simulink model "full_maneuver_platoon"  (R2022a)
settings: Solver=ode23t  StartTime=0.0  StopTime=300  FixedStep=0.1  MaxStep=0.01  RelTol=1e-3
InitFcn:
  | totalVehicles = 7;
  | if exist('vehStatesBus', 'var')==0
  | load vehBuses
  | end
  | if exist('vehErrorsBus', 'var')==0
  | load vehBuses
  | end
libraries: simulink x80, powerlib_meascontrol x16, autolibshared x7, dspsigops x4
(part 8 of 9)

== stateflow chart full_maneuver_platoon/p1/Lane Change Strategy/Strategy 1: synchronous/Chart ==
  state laneKeeping
    entry:
    maneuverState = 0;
    % canStartLaneChange = false;
  state generatingGapForMergingVehicle
    entry:
    maneuverState = 1;
    hasVirtualLeader = true;
  state gapClosing
    entry:
    maneuverState = 5;
    mustIncreaseGap = false;
  state generatingGap
    entry:
    maneuverState = 1;
    mustIncreaseGap = true;
    if positionInPlatoon == 1
    hasVirtualLeader = true;
    end
    if positionInPlatoon == length(platoonStates)
    hasVirtualFollower = true;
    end
  state waitingForGapClosing
    entry:
    maneuverState = 4;
    hasVirtualLeader = false;
  state laneChanging
    entry:
    maneuverState = 3;
    canStartLaneChange = true;
    hasVirtualFollower = false;
  state waitingForPlatoonSafeGap
    entry:
    maneuverState = 2;
  (default) -> laneKeeping
  laneKeeping -> generatingGapForMergingVehicle [order 1] : [gapRequest && platoonStates(end) <= 3]
  generatingGapForMergingVehicle -> laneKeeping : [platoonStates(end) > 3]
  gapClosing -> laneKeeping : [isGapClosed || (positionInPlatoon==1 ...
      | && realCACCstate~=1 && sum(platoonStates(2:end))==0 ...
      | && after(1, sec))]
  laneKeeping -> generatingGap [order 2] : [hasLaneChangeIntention && ~isLaneChangeDone ...
      |  && ((positionInPlatoon == 1) || (platoonStates(positionInPlatoon - 1)>1))]
  waitingForGapClosing -> gapClosing : [positionInPlatoon == length(platoonStates) || ...
      | platoonStates(positionInPlatoon + 1) == 0]
  laneChanging -> waitingForGapClosing : [isLaneChangeDone]
  generatingGap -> waitingForPlatoonSafeGap : [isLaneChangeSafe]
  waitingForPlatoonSafeGap -> laneChanging : [platoonStates(end)>1]
  data: gapRequest input; hasLaneChangeIntention input; maneuverState output uint8 =uint8(0); mustIncreaseGap output =false; positionInPlatoon input; platoonStates input; isLaneChangeDone input; isLaneChangeSafe input; canStartLaneChange output =false; hasVirtualLeader output =false; hasVirtualFollower output =false; isGapClosed input; realCACCstate input

== matlab function full_maneuver_platoon/p1/Lane Change Strategy/Strategy 1: synchronous/determine virtual leader idx/determineVirtualLeader ==
  data: nVehicles input; lcFlag input; virtualLeaderIdx output
function virtualLeaderIdx  = ...
    determineVirtualLeader(nVehicles, lcFlag)

% Strategy 'synchronous': all vehicles move together when gap fits the
% whole platoon
% Important assumption:
% The array of vehicles is ordered as [Ld, Fd, Lo, p1, ..., pN, Fo]

if ~lcFlag % gap generating vehicle
    virtualLeaderIdx = nVehicles-1; % last platoon vehicle
else % lane changing vehicle
    virtualLeaderIdx = 1;
end

end

== stateflow chart full_maneuver_platoon/p1/Lane Change Strategy/Strategy 2: leader first/Chart ==
  state laneKeeping
    entry:
    maneuverState = 0;
    % canStartLaneChange = false;
  state generatingGapForMergingVehicle
    entry:
    maneuverState = 1;
    hasVirtualLeader = true;
  state gapClosing
    entry:
    maneuverState = 5;
    mustIncreaseGap = false;
  state waitingLeaderLaneChange
    entry:
    maneuverState = 1;
    hasVirtualLeader = true;
  state waitingForGapClosing
    entry:
    maneuverState = 4;
    hasVirtualLeader = false;
  state laneChanging
    entry:
    maneuverState = 3;
    canStartLaneChange = true;
    hasVirtualFollower = false;
  state generatingGap
    entry:
    maneuverState = 2;
    mustIncreaseGap = true;
    hasVirtualLeader = true;
    hasVirtualFollower = true;
  (default) -> laneKeeping
  laneKeeping -> generatingGapForMergingVehicle [order 2] : [gapRequest && platoonStates(end) <= 3]
  gapClosing -> laneKeeping : [isGapClosed || (positionInPlatoon==1 ...
      | && realCACCstate~=1 && sum(platoonStates(2:end))==0 ...
      | && after(1, sec))]
  generatingGapForMergingVehicle -> laneKeeping : [platoonStates(end) > 3]
  laneKeeping -> waitingLeaderLaneChange [order 1] : [hasLaneChangeIntention && ~isLaneChangeDone ...
      |  && (positionInPlatoon == 1 || platoonStates(positionInPlatoon - 1) > 1)]
  waitingForGapClosing -> gapClosing : [true]
  waitingLeaderLaneChange -> generatingGap : [positionInPlatoon == 1 || platoonStates(positionInPlatoon - 1) > 4]
  laneChanging -> waitingForGapClosing : [isLaneChangeDone]
  generatingGap -> laneChanging : [isLaneChangeSafe]
  data: gapRequest input; hasLaneChangeIntention input; maneuverState output uint8 =uint8(0); mustIncreaseGap output =false; positionInPlatoon input; platoonStates input; isLaneChangeDone input; isLaneChangeSafe input; canStartLaneChange output =false; hasVirtualLeader output =false; hasVirtualFollower output =false; isGapClosed input; realCACCstate input

== matlab function full_maneuver_platoon/p1/Lane Change Strategy/Strategy 2: leader first/determine virtual leader idx/determineVirtualLeader ==
  data: nVehicles input; lcFlag input; virtualLeaderIdx output; posInPlatoon input
function virtualLeaderIdx  = ...
    determineVirtualLeader(nVehicles, lcFlag, posInPlatoon)

% Strategy: leader changes first 
% Important assumption:
% The array of vehicles is ordered as [Ld, Fd, Lo, p1, ..., pN, Fo]

if ~lcFlag% gap generating vehicle
    virtualLeaderIdx = nVehicles-1; % last platoon vehicle    
else % lane changing vehicle:  
    if posInPlatoon == 1
        virtualLeaderIdx = 1;
    else
        % all platoon vehicles adopt the real leading vehicle as
        % virtual leaders too
        virtualLeaderIdx = 3 + (posInPlatoon - 1);
    end
end

end

== stateflow chart full_maneuver_platoon/p1/Lane Change Strategy/Strategy 3: last first/Chart ==
  state generatingGapForMergingVehicle
    entry:
    maneuverState = 1;
    hasVirtualLeader = true;
  state laneKeeping
    entry:
    maneuverState = 0;
    % canStartLaneChange = false;
  state gapClosing
    entry:
    maneuverState = 5;
    hasVirtualLeader = false;
  state creatingGapForNextVehicle
    entry:
    maneuverState = 4;
    mustIncreaseGap = false;
  state generatingGap
    entry:
    maneuverState = 1;
    mustIncreaseGap = true;
    hasVirtualLeader = true;
    hasVirtualFollower = true;
  state laneChanging
    entry:
    maneuverState = 3;
    canStartLaneChange = true;
    hasVirtualFollower = false;
  (default) -> laneKeeping
  gapClosing -> laneKeeping : [isGapClosed || (positionInPlatoon==1 ...
      | && realCACCstate~=1 && sum(platoonStates(2:end))==0 ...
      | && after(1, sec))]
  laneKeeping -> generatingGapForMergingVehicle [order 2] : [gapRequest && platoonStates(end) <= 3]
  generatingGapForMergingVehicle -> laneKeeping : [platoonStates(end) > 3]
  laneKeeping -> generatingGap [order 1] : [hasLaneChangeIntention && ~isLaneChangeDone ...
      |  && (positionInPlatoon == length(platoonStates) || platoonStates(positionInPlatoon + 1) > 3)]
  creatingGapForNextVehicle -> gapClosing : [positionInPlatoon == 1 || ...
      | platoonStates(positionInPlatoon - 1) > 3]
  laneChanging -> creatingGapForNextVehicle : [isLaneChangeDone]
  generatingGap -> laneChanging : [isLaneChangeSafe]
  data: gapRequest input; hasLaneChangeIntention input; maneuverState output uint8 =uint8(0); mustIncreaseGap output =false; positionInPlatoon input; platoonStates input; isLaneChangeDone input; isLaneChangeSafe input; canStartLaneChange output =false; hasVirtualLeader output =false; hasVirtualFollower output =false; isGapClosed input; realCACCstate input

== matlab function full_maneuver_platoon/p1/Lane Change Strategy/Strategy 3: last first/determine virtual follower idx/determineVirtualFollower ==
  data: platoonSize input; posInPlatoon input; virtualFollowerIdx output
function virtualFollowerIdx  = ...
    determineVirtualFollower(platoonSize, posInPlatoon)

% Strategy 'lastFirst': last veh changes first and creates gap for leader
% Important assumption:
% The array of vehicles is ordered as [Ld, Fd, Lo, p1, ..., pN, Fo]

if posInPlatoon == platoonSize
    virtualFollowerIdx = 2;
else
    virtualFollowerIdx = 3 + (posInPlatoon + 1);
end

end

== matlab function full_maneuver_platoon/p1/Lane Change Strategy/Strategy 3: last first/determine virtual leader idx/determineVirtualLeader ==
  data: nVehicles input; lcFlag input; lcDone input; virtualLeaderIdx output; posInPlatoon input
function virtualLeaderIdx  = ...
    determineVirtualLeader(nVehicles, lcFlag, lcDone, posInPlatoon)

% Strategy 'lastFirst': last veh changes first and creates gap for leader
% Important assumption:
% The array of vehicles is ordered as [Ld, Fd, Lo, p1, ..., pN, Fo]

if ~lcFlag% gap generating vehicle
    virtualLeaderIdx = nVehicles-1; % last platoon vehicle
else % lane changing vehicle
    if ~lcDone
        virtualLeaderIdx = 1;
    else
        if posInPlatoon == 1
            virtualLeaderIdx = 1;
        else
            virtualLeaderIdx = 3 + (posInPlatoon - 1);
        end
    end
    
end

end

== stateflow chart full_maneuver_platoon/p1/Lane Change Strategy/Strategy 4: leader first invert/Chart ==
  state laneKeeping
    entry:
    maneuverState = 0;
    % canStartLaneChange = false;
  state generatingGapForMergingVehicle
    entry:
    maneuverState = 1;
    hasVirtualLeader = true;
  state gapClosing
    entry:
    maneuverState = 5;
    hasVirtualLeader = false;
  state creatingGapForNextVehicle
    entry:
    maneuverState = 4;
    mustIncreaseGap = false;
  state generatingGap
    entry:
    maneuverState = 1;
    mustIncreaseGap = true;
    hasVirtualLeader = true;
    hasVirtualFollower = true;
  state laneChanging
    entry:
    maneuverState = 3;
    canStartLaneChange = true;
    hasVirtualFollower = false;
  (default) -> laneKeeping
  gapClosing -> laneKeeping : [isGapClosed || (positionInPlatoon==length(platoonStates)...
      | && realCACCstate~=1 && sum(platoonStates(1:end-1))==0 ...
      | && after(1, sec))]
  laneKeeping -> generatingGapForMergingVehicle [order 2] : [gapRequest && platoonStates(1) <= 3]
  generatingGapForMergingVehicle -> laneKeeping : [platoonStates(1) > 3]
  laneKeeping -> generatingGap [order 1] : [hasLaneChangeIntention && ~isLaneChangeDone ...
      |  && (positionInPlatoon == 1 || platoonStates(positionInPlatoon - 1) > 3)]
  creatingGapForNextVehicle -> gapClosing : [positionInPlatoon == length(platoonStates) || ...
      | platoonStates(positionInPlatoon + 1) > 3]
  laneChanging -> creatingGapForNextVehicle : [isLaneChangeDone]
  generatingGap -> laneChanging : [isLaneChangeSafe]
  data: gapRequest input; hasLaneChangeIntention input; maneuverState output uint8 =uint8(0); mustIncreaseGap output =false; positionInPlatoon input; platoonStates input; isLaneChangeDone input; isLaneChangeSafe input; canStartLaneChange output =false; hasVirtualLeader output =false; hasVirtualFollower output =false; isGapClosed input; realCACCstate input

== matlab function full_maneuver_platoon/p1/Lane Change Strategy/Strategy 4: leader first invert/Subsystem/determineVirtualFollower ==
  data: posInPlatoon input; virtualFollowerIdx output
function virtualFollowerIdx  = ...
    determineVirtualFollower(posInPlatoon)

% Strategy 'leaderFirstInvert': leader changes first and creates gap for 
%next
% Important assumption:
% The array of vehicles is ordered as [Ld, Fd, Lo, p1, ..., pN, Fo]

if posInPlatoon == 1
    virtualFollowerIdx = 2;
else
    virtualFollowerIdx = 3 + (posInPlatoon - 1);
end


end

== matlab function full_maneuver_platoon/p1/Lane Change Strategy/Strategy 4: leader first invert/Subsystem1/determineVirtualLeader ==
  data: nVehicles input; lcFlag input; lcDone input; virtualLeaderIdx output; posInPlatoon input
function virtualLeaderIdx  = ...
    determineVirtualLeader(nVehicles, lcFlag, lcDone, posInPlatoon)

% Strategy 'leaderFirstInvert': leader changes first and creates gap for 
%next
% Important assumption:
% The array of vehicles is ordered as [Ld, Fd, Lo, p1, ..., pN, Fo]

platoonLength = nVehicles - 4;
if ~lcFlag% gap generating vehicle
    virtualLeaderIdx = 4; % first platoon vehicle
else % lane changing vehicle
    if ~lcDone
        virtualLeaderIdx = 1;
    else
        if posInPlatoon == platoonLength
            virtualLeaderIdx = 1;
        else
            virtualLeaderIdx = 3 + (posInPlatoon + 1);
        end
    end
end

end

== matlab function full_maneuver_platoon/p2/CACC destination lane/Virtual Vehicle Following/switch min vel/MATLAB Function ==
  data: h input; maxGap output; d0 input; vRef input; ev input; ehDot input; ea input; Kp parameter; Kd parameter; Ka parameter; Kdd parameter
function maxGap = followingGapThreshold(h, d0, vRef, ev, ehDot, ea, Kp, Kd, Ka, Kdd)

maxGap = h*vRef + d0 - 1/Kp*(Kd*ev + Kdd*ehDot + Ka*ea);

== matlab function full_maneuver_platoon/p2/CACC origin lane/switch free flow/MATLAB Function ==
  data: h input; maxGap output; d0 input; vRef input; ev input; ehDot input; ea input; Kp parameter; Kd parameter; Ka parameter; Kdd parameter
function maxGap = followingGapThreshold(h, d0, vRef, ev, ehDot, ea, Kp, Kd, Ka, Kdd)

maxGap = h*vRef + d0 - 1/Kp*(Kd*ev + Kdd*ehDot + Ka*ea);

== matlab function full_maneuver_platoon/p2/Find Leader/Subsystem/MATLAB Function ==
  data: ego input Bus: vehStatesBus; allVehicles input; leaderIdx output
function leaderIdx  = findLeader(ego, allVehicles)

nv = length(allVehicles);

leaderIdx = nv + 1;
leaderX = ego.X + 10^3;
% For non lane changing vehicles, the leader is whoever is longitudinally
% closer and with any part of the body in the same lane.
% 1.8m (half lane) + 0.9m (half veh width)
for n = 1:nv
    if allVehicles(n).X > ego.X
        if abs(allVehicles(n).Y - ego.Y) <= 2.7 ...
                && allVehicles(n).X < leaderX
            leaderIdx = n;
            leaderX = allVehicles(n).X;
        end
    end
end

== stateflow chart full_maneuver_platoon/p2/Lane Change Strategy/Strategy 1: synchronous/Chart ==
  state laneKeeping
    entry:
    maneuverState = 0;
    % canStartLaneChange = false;
  state generatingGapForMergingVehicle
    entry:
    maneuverState = 1;
    hasVirtualLeader = true;
  state gapClosing
    entry:
    maneuverState = 5;
    mustIncreaseGap = false;
  state generatingGap
    entry:
    maneuverState = 1;
    mustIncreaseGap = true;
    if positionInPlatoon == 1
    hasVirtualLeader = true;
    end
    if positionInPlatoon == length(platoonStates)
    hasVirtualFollower = true;
    end
  state waitingForGapClosing
    entry:
    maneuverState = 4;
    hasVirtualLeader = false;
  state laneChanging
    entry:
    maneuverState = 3;
    canStartLaneChange = true;
    hasVirtualFollower = false;
  state waitingForPlatoonSafeGap
    entry:
    maneuverState = 2;
  (default) -> laneKeeping
  laneKeeping -> generatingGapForMergingVehicle [order 1] : [gapRequest && platoonStates(end) <= 3]
  generatingGapForMergingVehicle -> laneKeeping : [platoonStates(end) > 3]
  gapClosing -> laneKeeping : [isGapClosed || (positionInPlatoon==1 ...
      | && realCACCstate~=1 && sum(platoonStates(2:end))==0 ...
      | && after(1, sec))]
  laneKeeping -> generatingGap [order 2] : [hasLaneChangeIntention && ~isLaneChangeDone ...
      |  && ((positionInPlatoon == 1) || (platoonStates(positionInPlatoon - 1)>1))]
  waitingForGapClosing -> gapClosing : [positionInPlatoon == length(platoonStates) || ...
      | platoonStates(positionInPlatoon + 1) == 0]
  laneChanging -> waitingForGapClosing : [isLaneChangeDone]
  generatingGap -> waitingForPlatoonSafeGap : [isLaneChangeSafe]
  waitingForPlatoonSafeGap -> laneChanging : [platoonStates(end)>1]
  data: gapRequest input; hasLaneChangeIntention input; maneuverState output uint8 =uint8(0); mustIncreaseGap output =false; positionInPlatoon input; platoonStates input; isLaneChangeDone input; isLaneChangeSafe input; canStartLaneChange output =false; hasVirtualLeader output =false; hasVirtualFollower output =false; isGapClosed input; realCACCstate input

== matlab function full_maneuver_platoon/p2/Lane Change Strategy/Strategy 1: synchronous/determine virtual leader idx/determineVirtualLeader ==
  data: nVehicles input; lcFlag input; virtualLeaderIdx output
function virtualLeaderIdx  = ...
    determineVirtualLeader(nVehicles, lcFlag)

% Strategy 'synchronous': all vehicles move together when gap fits the
% whole platoon
% Important assumption:
% The array of vehicles is ordered as [Ld, Fd, Lo, p1, ..., pN, Fo]

if ~lcFlag % gap generating vehicle
    virtualLeaderIdx = nVehicles-1; % last platoon vehicle
else % lane changing vehicle
    virtualLeaderIdx = 1;
end

end

== stateflow chart full_maneuver_platoon/p2/Lane Change Strategy/Strategy 2: leader first/Chart ==
  state laneKeeping
    entry:
    maneuverState = 0;
    % canStartLaneChange = false;
  state generatingGapForMergingVehicle
    entry:
    maneuverState = 1;
    hasVirtualLeader = true;
  state gapClosing
    entry:
    maneuverState = 5;
    mustIncreaseGap = false;
  state waitingLeaderLaneChange
    entry:
    maneuverState = 1;
    hasVirtualLeader = true;
  state waitingForGapClosing
    entry:
    maneuverState = 4;
    hasVirtualLeader = false;
  state laneChanging
    entry:
    maneuverState = 3;
    canStartLaneChange = true;
    hasVirtualFollower = false;
  state generatingGap
    entry:
    maneuverState = 2;
    mustIncreaseGap = true;
    hasVirtualLeader = true;
    hasVirtualFollower = true;
  (default) -> laneKeeping
  laneKeeping -> generatingGapForMergingVehicle [order 2] : [gapRequest && platoonStates(end) <= 3]
  gapClosing -> laneKeeping : [isGapClosed || (positionInPlatoon==1 ...
      | && realCACCstate~=1 && sum(platoonStates(2:end))==0 ...
      | && after(1, sec))]
  generatingGapForMergingVehicle -> laneKeeping : [platoonStates(end) > 3]
  laneKeeping -> waitingLeaderLaneChange [order 1] : [hasLaneChangeIntention && ~isLaneChangeDone ...
      |  && (positionInPlatoon == 1 || platoonStates(positionInPlatoon - 1) > 1)]
  waitingForGapClosing -> gapClosing : [true]
  waitingLeaderLaneChange -> generatingGap : [positionInPlatoon == 1 || platoonStates(positionInPlatoon - 1) > 4]
  laneChanging -> waitingForGapClosing : [isLaneChangeDone]
  generatingGap -> laneChanging : [isLaneChangeSafe]
  data: gapRequest input; hasLaneChangeIntention input; maneuverState output uint8 =uint8(0); mustIncreaseGap output =false; positionInPlatoon input; platoonStates input; isLaneChangeDone input; isLaneChangeSafe input; canStartLaneChange output =false; hasVirtualLeader output =false; hasVirtualFollower output =false; isGapClosed input; realCACCstate input

== matlab function full_maneuver_platoon/p2/Lane Change Strategy/Strategy 2: leader first/determine virtual leader idx/determineVirtualLeader ==
  data: nVehicles input; lcFlag input; virtualLeaderIdx output; posInPlatoon input
function virtualLeaderIdx  = ...
    determineVirtualLeader(nVehicles, lcFlag, posInPlatoon)

% Strategy: leader changes first 
% Important assumption:
% The array of vehicles is ordered as [Ld, Fd, Lo, p1, ..., pN, Fo]

if ~lcFlag% gap generating vehicle
    virtualLeaderIdx = nVehicles-1; % last platoon vehicle    
else % lane changing vehicle:  
    if posInPlatoon == 1
        virtualLeaderIdx = 1;
    else
        % all platoon vehicles adopt the real leading vehicle as
        % virtual leaders too
        virtualLeaderIdx = 3 + (posInPlatoon - 1);
    end
end

end

== stateflow chart full_maneuver_platoon/p2/Lane Change Strategy/Strategy 3: last first/Chart ==
  state generatingGapForMergingVehicle
    entry:
    maneuverState = 1;
    hasVirtualLeader = true;
  state laneKeeping
    entry:
    maneuverState = 0;
    % canStartLaneChange = false;
  state gapClosing
    entry:
    maneuverState = 5;
    hasVirtualLeader = false;
  state creatingGapForNextVehicle
    entry:
    maneuverState = 4;
    mustIncreaseGap = false;
  state generatingGap
    entry:
    maneuverState = 1;
    mustIncreaseGap = true;
    hasVirtualLeader = true;
    hasVirtualFollower = true;
  state laneChanging
    entry:
    maneuverState = 3;
    canStartLaneChange = true;
    hasVirtualFollower = false;
  (default) -> laneKeeping
  gapClosing -> laneKeeping : [isGapClosed || (positionInPlatoon==1 ...
      | && realCACCstate~=1 && sum(platoonStates(2:end))==0 ...
      | && after(1, sec))]
  laneKeeping -> generatingGapForMergingVehicle [order 2] : [gapRequest && platoonStates(end) <= 3]
  generatingGapForMergingVehicle -> laneKeeping : [platoonStates(end) > 3]
  laneKeeping -> generatingGap [order 1] : [hasLaneChangeIntention && ~isLaneChangeDone ...
      |  && (positionInPlatoon == length(platoonStates) || platoonStates(positionInPlatoon + 1) > 3)]
  creatingGapForNextVehicle -> gapClosing : [positionInPlatoon == 1 || ...
      | platoonStates(positionInPlatoon - 1) > 3]
  laneChanging -> creatingGapForNextVehicle : [isLaneChangeDone]
  generatingGap -> laneChanging : [isLaneChangeSafe]
  data: gapRequest input; hasLaneChangeIntention input; maneuverState output uint8 =uint8(0); mustIncreaseGap output =false; positionInPlatoon input; platoonStates input; isLaneChangeDone input; isLaneChangeSafe input; canStartLaneChange output =false; hasVirtualLeader output =false; hasVirtualFollower output =false; isGapClosed input; realCACCstate input

== matlab function full_maneuver_platoon/Lo/CACC origin lane/Controller Real Leader/switch free flow/MATLAB Function ==
  data: h input; maxGap output; d0 input; vRef input; ev input; ehDot input; ea input; Kp parameter; Kd parameter; Ka parameter; Kdd parameter
function maxGap = followingGapThreshold(h, d0, vRef, ev, ehDot, ea, Kp, Kd, Ka, Kdd)

maxGap = h*vRef + d0 - 1/Kp*(Kd*ev + Kdd*ehDot + Ka*ea);

== matlab function full_maneuver_platoon/Ld/findLeader/Subsystem/MATLAB Function ==
  data: ego input Bus: vehStatesBus; allVehicles input; leaderIdx output
function leaderIdx  = findLeader(ego, allVehicles)

nv = length(allVehicles);

leaderIdx = nv + 1;
leaderX = ego.X + 10^3;
% For non lane changing vehicles, the leader is whoever is longitudinally
% closer and with any part of the body in the same lane.
% 1.8m (half lane) + 0.9m (half veh width)
for n = 1:nv
    if allVehicles(n).X>ego.X
        if abs(allVehicles(n).Y - ego.Y)<=2.7 && allVehicles(n).X<leaderX
            leaderIdx = n;
            leaderX = allVehicles(n).X;
        end
    end
end

== matlab function full_maneuver_platoon/Lo/findLeader/Subsystem/MATLAB Function ==
  data: ego input Bus: vehStatesBus; allVehicles input; leaderIdx output
function leaderIdx  = findLeader(ego, allVehicles)

nv = length(allVehicles);

leaderIdx = nv + 1;
leaderX = ego.X + 10^3;
% For non lane changing vehicles, the leader is whoever is longitudinally
% closer and with any part of the body in the same lane.
% 1.8m (half lane) + 0.9m (half veh width)
for n = 1:nv
    if allVehicles(n).X>ego.X
        if abs(allVehicles(n).Y - ego.Y)<=2.7 && allVehicles(n).X<leaderX
            leaderIdx = n;
            leaderX = allVehicles(n).X;
        end
    end
end

== matlab function full_maneuver_platoon/p2/Lane Change Strategy/Strategy 3: last first/determine virtual follower idx/determineVirtualFollower ==
  data: platoonSize input; posInPlatoon input; virtualFollowerIdx output
function virtualFollowerIdx  = ...
    determineVirtualFollower(platoonSize, posInPlatoon)

% Strategy 'lastFirst': last veh changes first and creates gap for leader
% Important assumption:
% The array of vehicles is ordered as [Ld, Fd, Lo, p1, ..., pN, Fo]

if posInPlatoon == platoonSize
    virtualFollowerIdx = 2;
else
    virtualFollowerIdx = 3 + (posInPlatoon + 1);
end

end

== matlab function full_maneuver_platoon/p1/CACC destination lane/Virtual Vehicle Following/switch min vel/MATLAB Function ==
  data: h input; maxGap output; d0 input; vRef input; ev input; ehDot input; ea input; Kp parameter; Kd parameter; Ka parameter; Kdd parameter
function maxGap = followingGapThreshold(h, d0, vRef, ev, ehDot, ea, Kp, Kd, Ka, Kdd)

maxGap = h*vRef + d0 - 1/Kp*(Kd*ev + Kdd*ehDot + Ka*ea);

== matlab function full_maneuver_platoon/p2/Lane Change Strategy/Strategy 3: last first/determine virtual leader idx/determineVirtualLeader ==
  data: nVehicles input; lcFlag input; lcDone input; virtualLeaderIdx output; posInPlatoon input
function virtualLeaderIdx  = ...
    determineVirtualLeader(nVehicles, lcFlag, lcDone, posInPlatoon)

% Strategy 'lastFirst': last veh changes first and creates gap for leader
% Important assumption:
% The array of vehicles is ordered as [Ld, Fd, Lo, p1, ..., pN, Fo]

if ~lcFlag% gap generating vehicle
    virtualLeaderIdx = nVehicles-1; % last platoon vehicle
else % lane changing vehicle
    if ~lcDone
        virtualLeaderIdx = 1;
    else
        if posInPlatoon == 1
            virtualLeaderIdx = 1;
        else
            virtualLeaderIdx = 3 + (posInPlatoon - 1);
        end
    end
    
end

end

== stateflow chart full_maneuver_platoon/p2/Lane Change Strategy/Strategy 4: leader first invert/Chart ==
  state laneKeeping
    entry:
    maneuverState = 0;
    % canStartLaneChange = false;
  state generatingGapForMergingVehicle
    entry:
    maneuverState = 1;
    hasVirtualLeader = true;
  state gapClosing
    entry:
    maneuverState = 5;
    hasVirtualLeader = false;
  state creatingGapForNextVehicle
    entry:
    maneuverState = 4;
    mustIncreaseGap = false;
  state generatingGap
    entry:
    maneuverState = 1;
    mustIncreaseGap = true;
    hasVirtualLeader = true;
    hasVirtualFollower = true;
  state laneChanging
    entry:
    maneuverState = 3;
    canStartLaneChange = true;
    hasVirtualFollower = false;
  (default) -> laneKeeping
  gapClosing -> laneKeeping : [isGapClosed || (positionInPlatoon==length(platoonStates)...
      | && realCACCstate~=1 && sum(platoonStates(1:end-1))==0 ...
      | && after(1, sec))]
  laneKeeping -> generatingGapForMergingVehicle [order 2] : [gapRequest && platoonStates(1) <= 3]
  generatingGapForMergingVehicle -> laneKeeping : [platoonStates(1) > 3]
  laneKeeping -> generatingGap [order 1] : [hasLaneChangeIntention && ~isLaneChangeDone ...
      |  && (positionInPlatoon == 1 || platoonStates(positionInPlatoon - 1) > 3)]
  creatingGapForNextVehicle -> gapClosing : [positionInPlatoon == length(platoonStates) || ...
      | platoonStates(positionInPlatoon + 1) > 3]
  laneChanging -> creatingGapForNextVehicle : [isLaneChangeDone]
  generatingGap -> laneChanging : [isLaneChangeSafe]
  data: gapRequest input; hasLaneChangeIntention input; maneuverState output uint8 =uint8(0); mustIncreaseGap output =false; positionInPlatoon input; platoonStates input; isLaneChangeDone input; isLaneChangeSafe input; canStartLaneChange output =false; hasVirtualLeader output =false; hasVirtualFollower output =false; isGapClosed input; realCACCstate input

== matlab function full_maneuver_platoon/p2/Lane Change Strategy/Strategy 4: leader first invert/Subsystem/determineVirtualFollower ==
  data: posInPlatoon input; virtualFollowerIdx output
function virtualFollowerIdx  = ...
    determineVirtualFollower(posInPlatoon)

% Strategy 'leaderFirstInvert': leader changes first and creates gap for 
%next
% Important assumption:
% The array of vehicles is ordered as [Ld, Fd, Lo, p1, ..., pN, Fo]

if posInPlatoon == 1
    virtualFollowerIdx = 2;
else
    virtualFollowerIdx = 3 + (posInPlatoon - 1);
end


end

== matlab function full_maneuver_platoon/p2/Lane Change Strategy/Strategy 4: leader first invert/Subsystem1/determineVirtualLeader ==
  data: nVehicles input; lcFlag input; lcDone input; virtualLeaderIdx output; posInPlatoon input
function virtualLeaderIdx  = ...
    determineVirtualLeader(nVehicles, lcFlag, lcDone, posInPlatoon)

% Strategy 'leaderFirstInvert': leader changes first and creates gap for 
%next
% Important assumption:
% The array of vehicles is ordered as [Ld, Fd, Lo, p1, ..., pN, Fo]

platoonLength = nVehicles - 4;
if ~lcFlag% gap generating vehicle
    virtualLeaderIdx = 4; % first platoon vehicle
else % lane changing vehicle
    if ~lcDone
        virtualLeaderIdx = 1;
    else
        if posInPlatoon == platoonLength
            virtualLeaderIdx = 1;
        else
            virtualLeaderIdx = 3 + (posInPlatoon + 1);
        end
    end
end

end

== matlab function full_maneuver_platoon/p3/CACC destination lane/Virtual Vehicle Following/switch min vel/MATLAB Function ==
  data: h input; maxGap output; d0 input; vRef input; ev input; ehDot input; ea input; Kp parameter; Kd parameter; Ka parameter; Kdd parameter
function maxGap = followingGapThreshold(h, d0, vRef, ev, ehDot, ea, Kp, Kd, Ka, Kdd)

maxGap = h*vRef + d0 - 1/Kp*(Kd*ev + Kdd*ehDot + Ka*ea);

== matlab function full_maneuver_platoon/p3/CACC origin lane/switch free flow/MATLAB Function ==
  data: h input; maxGap output; d0 input; vRef input; ev input; ehDot input; ea input; Kp parameter; Kd parameter; Ka parameter; Kdd parameter
function maxGap = followingGapThreshold(h, d0, vRef, ev, ehDot, ea, Kp, Kd, Ka, Kdd)

maxGap = h*vRef + d0 - 1/Kp*(Kd*ev + Kdd*ehDot + Ka*ea);

== matlab function full_maneuver_platoon/p3/Find Leader/Subsystem/MATLAB Function ==
  data: ego input Bus: vehStatesBus; allVehicles input; leaderIdx output
function leaderIdx  = findLeader(ego, allVehicles)

nv = length(allVehicles);

leaderIdx = nv + 1;
leaderX = ego.X + 10^3;
% For non lane changing vehicles, the leader is whoever is longitudinally
% closer and with any part of the body in the same lane.
% 1.8m (half lane) + 0.9m (half veh width)
for n = 1:nv
    if allVehicles(n).X > ego.X
        if abs(allVehicles(n).Y - ego.Y) <= 2.7 ...
                && allVehicles(n).X < leaderX
            leaderIdx = n;
            leaderX = allVehicles(n).X;
        end
    end
end

== stateflow chart full_maneuver_platoon/p3/Lane Change Strategy/Strategy 1: synchronous/Chart ==
  state laneKeeping
    entry:
    maneuverState = 0;
    % canStartLaneChange = false;
  state generatingGapForMergingVehicle
    entry:
    maneuverState = 1;
    hasVirtualLeader = true;
  state gapClosing
    entry:
    maneuverState = 5;
    mustIncreaseGap = false;
  state generatingGap
    entry:
    maneuverState = 1;
    mustIncreaseGap = true;
    if positionInPlatoon == 1
    hasVirtualLeader = true;
    end
    if positionInPlatoon == length(platoonStates)
    hasVirtualFollower = true;
    end
  state waitingForGapClosing
    entry:
    maneuverState = 4;
    hasVirtualLeader = false;
  state laneChanging
    entry:
    maneuverState = 3;
    canStartLaneChange = true;
    hasVirtualFollower = false;
  state waitingForPlatoonSafeGap
    entry:
    maneuverState = 2;
  (default) -> laneKeeping
  laneKeeping -> generatingGapForMergingVehicle [order 1] : [gapRequest && platoonStates(end) <= 3]
  generatingGapForMergingVehicle -> laneKeeping : [platoonStates(end) > 3]
  gapClosing -> laneKeeping : [isGapClosed || (positionInPlatoon==1 ...
      | && realCACCstate~=1 && sum(platoonStates(2:end))==0 ...
      | && after(1, sec))]
  laneKeeping -> generatingGap [order 2] : [hasLaneChangeIntention && ~isLaneChangeDone ...
      |  && ((positionInPlatoon == 1) || (platoonStates(positionInPlatoon - 1)>1))]
  waitingForGapClosing -> gapClosing : [positionInPlatoon == length(platoonStates) || ...
      | platoonStates(positionInPlatoon + 1) == 0]
  laneChanging -> waitingForGapClosing : [isLaneChangeDone]
  generatingGap -> waitingForPlatoonSafeGap : [isLaneChangeSafe]
  waitingForPlatoonSafeGap -> laneChanging : [platoonStates(end)>1]
  data: gapRequest input; hasLaneChangeIntention input; maneuverState output uint8 =uint8(0); mustIncreaseGap output =false; positionInPlatoon input; platoonStates input; isLaneChangeDone input; isLaneChangeSafe input; canStartLaneChange output =false; hasVirtualLeader output =false; hasVirtualFollower output =false; isGapClosed input; realCACCstate input

== matlab function full_maneuver_platoon/Fo/CACC origin lane/Controller Real Leader/switch free flow/MATLAB Function ==
  data: h input; maxGap output; d0 input; vRef input; ev input; ehDot input; ea input; Kp parameter; Kd parameter; Ka parameter; Kdd parameter
function maxGap = followingGapThreshold(h, d0, vRef, ev, ehDot, ea, Kp, Kd, Ka, Kdd)

maxGap = h*vRef + d0 - 1/Kp*(Kd*ev + Kdd*ehDot + Ka*ea);

== matlab function full_maneuver_platoon/p3/Lane Change Strategy/Strategy 1: synchronous/determine virtual leader idx/determineVirtualLeader ==
  data: nVehicles input; lcFlag input; virtualLeaderIdx output
function virtualLeaderIdx  = ...
    determineVirtualLeader(nVehicles, lcFlag)

% Strategy 'synchronous': all vehicles move together when gap fits the
% whole platoon
% Important assumption:
% The array of vehicles is ordered as [Ld, Fd, Lo, p1, ..., pN, Fo]

if ~lcFlag % gap generating vehicle
    virtualLeaderIdx = nVehicles-1; % last platoon vehicle
else % lane changing vehicle
    virtualLeaderIdx = 1;
end

end

== stateflow chart full_maneuver_platoon/p3/Lane Change Strategy/Strategy 2: leader first/Chart ==
  state laneKeeping
    entry:
    maneuverState = 0;
    % canStartLaneChange = false;
  state generatingGapForMergingVehicle
    entry:
    maneuverState = 1;
    hasVirtualLeader = true;
  state gapClosing
    entry:
    maneuverState = 5;
    mustIncreaseGap = false;
  state waitingLeaderLaneChange
    entry:
    maneuverState = 1;
    hasVirtualLeader = true;
  state waitingForGapClosing
    entry:
    maneuverState = 4;
    hasVirtualLeader = false;
  state laneChanging
    entry:
    maneuverState = 3;
    canStartLaneChange = true;
    hasVirtualFollower = false;
  state generatingGap
    entry:
    maneuverState = 2;
    mustIncreaseGap = true;
    hasVirtualLeader = true;
    hasVirtualFollower = true;
  (default) -> laneKeeping
  laneKeeping -> generatingGapForMergingVehicle [order 2] : [gapRequest && platoonStates(end) <= 3]
  gapClosing -> laneKeeping : [isGapClosed || (positionInPlatoon==1 ...
      | && realCACCstate~=1 && sum(platoonStates(2:end))==0 ...
      | && after(1, sec))]
  generatingGapForMergingVehicle -> laneKeeping : [platoonStates(end) > 3]
  laneKeeping -> waitingLeaderLaneChange [order 1] : [hasLaneChangeIntention && ~isLaneChangeDone ...
      |  && (positionInPlatoon == 1 || platoonStates(positionInPlatoon - 1) > 1)]
  waitingForGapClosing -> gapClosing : [true]
  waitingLeaderLaneChange -> generatingGap : [positionInPlatoon == 1 || platoonStates(positionInPlatoon - 1) > 4]
  laneChanging -> waitingForGapClosing : [isLaneChangeDone]
  generatingGap -> laneChanging : [isLaneChangeSafe]
  data: gapRequest input; hasLaneChangeIntention input; maneuverState output uint8 =uint8(0); mustIncreaseGap output =false; positionInPlatoon input; platoonStates input; isLaneChangeDone input; isLaneChangeSafe input; canStartLaneChange output =false; hasVirtualLeader output =false; hasVirtualFollower output =false; isGapClosed input; realCACCstate input

== matlab function full_maneuver_platoon/p1/CACC origin lane/switch free flow/MATLAB Function ==
  data: h input; maxGap output; d0 input; vRef input; ev input; ehDot input; ea input; Kp parameter; Kd parameter; Ka parameter; Kdd parameter
function maxGap = followingGapThreshold(h, d0, vRef, ev, ehDot, ea, Kp, Kd, Ka, Kdd)

maxGap = h*vRef + d0 - 1/Kp*(Kd*ev + Kdd*ehDot + Ka*ea);

== matlab function full_maneuver_platoon/p3/Lane Change Strategy/Strategy 2: leader first/determine virtual leader idx/determineVirtualLeader ==
  data: nVehicles input; lcFlag input; virtualLeaderIdx output; posInPlatoon input
function virtualLeaderIdx  = ...
    determineVirtualLeader(nVehicles, lcFlag, posInPlatoon)

% Strategy: leader changes first 
% Important assumption:
% The array of vehicles is ordered as [Ld, Fd, Lo, p1, ..., pN, Fo]

if ~lcFlag% gap generating vehicle
    virtualLeaderIdx = nVehicles-1; % last platoon vehicle    
else % lane changing vehicle:  
    if posInPlatoon == 1
        virtualLeaderIdx = 1;
    else
        % all platoon vehicles adopt the real leading vehicle as
        % virtual leaders too
        virtualLeaderIdx = 3 + (posInPlatoon - 1);
    end
end

end

== stateflow chart full_maneuver_platoon/p3/Lane Change Strategy/Strategy 3: last first/Chart ==
  state generatingGapForMergingVehicle
    entry:
    maneuverState = 1;
    hasVirtualLeader = true;
  state laneKeeping
    entry:
    maneuverState = 0;
    % canStartLaneChange = false;
  state gapClosing
    entry:
    maneuverState = 5;
    hasVirtualLeader = false;
  state creatingGapForNextVehicle
    entry:
    maneuverState = 4;
    mustIncreaseGap = false;
  state generatingGap
    entry:
    maneuverState = 1;
    mustIncreaseGap = true;
    hasVirtualLeader = true;
    hasVirtualFollower = true;
  state laneChanging
    entry:
    maneuverState = 3;
    canStartLaneChange = true;
    hasVirtualFollower = false;
  (default) -> laneKeeping
  gapClosing -> laneKeeping : [isGapClosed || (positionInPlatoon==1 ...
      | && realCACCstate~=1 && sum(platoonStates(2:end))==0 ...
      | && after(1, sec))]
  laneKeeping -> generatingGapForMergingVehicle [order 2] : [gapRequest && platoonStates(end) <= 3]
  generatingGapForMergingVehicle -> laneKeeping : [platoonStates(end) > 3]
  laneKeeping -> generatingGap [order 1] : [hasLaneChangeIntention && ~isLaneChangeDone ...
      |  && (positionInPlatoon == length(platoonStates) || platoonStates(positionInPlatoon + 1) > 3)]
  creatingGapForNextVehicle -> gapClosing : [positionInPlatoon == 1 || ...
      | platoonStates(positionInPlatoon - 1) > 3]
  laneChanging -> creatingGapForNextVehicle : [isLaneChangeDone]
  generatingGap -> laneChanging : [isLaneChangeSafe]
  data: gapRequest input; hasLaneChangeIntention input; maneuverState output uint8 =uint8(0); mustIncreaseGap output =false; positionInPlatoon input; platoonStates input; isLaneChangeDone input; isLaneChangeSafe input; canStartLaneChange output =false; hasVirtualLeader output =false; hasVirtualFollower output =false; isGapClosed input; realCACCstate input

== matlab function full_maneuver_platoon/p3/Lane Change Strategy/Strategy 3: last first/determine virtual follower idx/determineVirtualFollower ==
  data: platoonSize input; posInPlatoon input; virtualFollowerIdx output
function virtualFollowerIdx  = ...
    determineVirtualFollower(platoonSize, posInPlatoon)

% Strategy 'lastFirst': last veh changes first and creates gap for leader
% Important assumption:
% The array of vehicles is ordered as [Ld, Fd, Lo, p1, ..., pN, Fo]

if posInPlatoon == platoonSize
    virtualFollowerIdx = 2;
else
    virtualFollowerIdx = 3 + (posInPlatoon + 1);
end

end

== matlab function full_maneuver_platoon/p3/Lane Change Strategy/Strategy 3: last first/determine virtual leader idx/determineVirtualLeader ==
  data: nVehicles input; lcFlag input; lcDone input; virtualLeaderIdx output; posInPlatoon input
function virtualLeaderIdx  = ...
    determineVirtualLeader(nVehicles, lcFlag, lcDone, posInPlatoon)

% Strategy 'lastFirst': last veh changes first and creates gap for leader
% Important assumption:
% The array of vehicles is ordered as [Ld, Fd, Lo, p1, ..., pN, Fo]

if ~lcFlag% gap generating vehicle
    virtualLeaderIdx = nVehicles-1; % last platoon vehicle
else % lane changing vehicle
    if ~lcDone
        virtualLeaderIdx = 1;
    else
        if posInPlatoon == 1
            virtualLeaderIdx = 1;
        else
            virtualLeaderIdx = 3 + (posInPlatoon - 1);
        end
    end
    
end

end

== stateflow chart full_maneuver_platoon/p3/Lane Change Strategy/Strategy 4: leader first invert/Chart ==
  state laneKeeping
    entry:
    maneuverState = 0;
    % canStartLaneChange = false;
  state generatingGapForMergingVehicle
    entry:
    maneuverState = 1;
    hasVirtualLeader = true;
  state gapClosing
    entry:
    maneuverState = 5;
    hasVirtualLeader = false;
  state creatingGapForNextVehicle
    entry:
    maneuverState = 4;
    mustIncreaseGap = false;
  state generatingGap
    entry:
    maneuverState = 1;
    mustIncreaseGap = true;
    hasVirtualLeader = true;
    hasVirtualFollower = true;
  state laneChanging
    entry:
    maneuverState = 3;
    canStartLaneChange = true;
    hasVirtualFollower = false;
  (default) -> laneKeeping
  gapClosing -> laneKeeping : [isGapClosed || (positionInPlatoon==length(platoonStates)...
      | && realCACCstate~=1 && sum(platoonStates(1:end-1))==0 ...
      | && after(1, sec))]
  laneKeeping -> generatingGapForMergingVehicle [order 2] : [gapRequest && platoonStates(1) <= 3]
  generatingGapForMergingVehicle -> laneKeeping : [platoonStates(1) > 3]
  laneKeeping -> generatingGap [order 1] : [hasLaneChangeIntention && ~isLaneChangeDone ...
      |  && (positionInPlatoon == 1 || platoonStates(positionInPlatoon - 1) > 3)]
  creatingGapForNextVehicle -> gapClosing : [positionInPlatoon == length(platoonStates) || ...
      | platoonStates(positionInPlatoon + 1) > 3]
  laneChanging -> creatingGapForNextVehicle : [isLaneChangeDone]
  generatingGap -> laneChanging : [isLaneChangeSafe]
  data: gapRequest input; hasLaneChangeIntention input; maneuverState output uint8 =uint8(0); mustIncreaseGap output =false; positionInPlatoon input; platoonStates input; isLaneChangeDone input; isLaneChangeSafe input; canStartLaneChange output =false; hasVirtualLeader output =false; hasVirtualFollower output =false; isGapClosed input; realCACCstate input

== matlab function full_maneuver_platoon/p3/Lane Change Strategy/Strategy 4: leader first invert/Subsystem/determineVirtualFollower ==
  data: posInPlatoon input; virtualFollowerIdx output
function virtualFollowerIdx  = ...
    determineVirtualFollower(posInPlatoon)

% Strategy 'leaderFirstInvert': leader changes first and creates gap for 
%next
% Important assumption:
% The array of vehicles is ordered as [Ld, Fd, Lo, p1, ..., pN, Fo]

if posInPlatoon == 1
    virtualFollowerIdx = 2;
else
    virtualFollowerIdx = 3 + (posInPlatoon - 1);
end


end

== matlab function full_maneuver_platoon/p3/Lane Change Strategy/Strategy 4: leader first invert/Subsystem1/determineVirtualLeader ==
  data: nVehicles input; lcFlag input; lcDone input; virtualLeaderIdx output; posInPlatoon input
function virtualLeaderIdx  = ...
    determineVirtualLeader(nVehicles, lcFlag, lcDone, posInPlatoon)

% Strategy 'leaderFirstInvert': leader changes first and creates gap for 
%next
% Important assumption:
% The array of vehicles is ordered as [Ld, Fd, Lo, p1, ..., pN, Fo]

platoonLength = nVehicles - 4;
if ~lcFlag% gap generating vehicle
    virtualLeaderIdx = 4; % first platoon vehicle
else % lane changing vehicle
    if ~lcDone
        virtualLeaderIdx = 1;
    else
        if posInPlatoon == platoonLength
            virtualLeaderIdx = 1;
        else
            virtualLeaderIdx = 3 + (posInPlatoon + 1);
        end
    end
end

end

== matlab function full_maneuver_platoon/Fd/CACC destination lane/Virtual Vehicle Following/switch min vel/MATLAB Function ==
  data: h input; maxGap output; d0 input; vRef input; ev input; ehDot input; ea input; Kp parameter; Kd parameter; Ka parameter; Kdd parameter
function maxGap = followingGapThreshold(h, d0, vRef, ev, ehDot, ea, Kp, Kd, Ka, Kdd)

maxGap = h*vRef + d0 - 1/Kp*(Kd*ev + Kdd*ehDot + Ka*ea);

== matlab function full_maneuver_platoon/Fd/CACC origin lane/Controller Real Leader/switch free flow/MATLAB Function ==
  data: h input; maxGap output; d0 input; vRef input; ev input; ehDot input; ea input; Kp parameter; Kd parameter; Ka parameter; Kdd parameter
function maxGap = followingGapThreshold(h, d0, vRef, ev, ehDot, ea, Kp, Kd, Ka, Kdd)

maxGap = h*vRef + d0 - 1/Kp*(Kd*ev + Kdd*ehDot + Ka*ea);

== matlab function full_maneuver_platoon/Fd/Find Leader/Subsystem/MATLAB Function ==
  data: ego input Bus: vehStatesBus; allVehicles input; leaderIdx output
function leaderIdx  = findLeader(ego, allVehicles)

nv = length(allVehicles);

leaderIdx = nv + 1;
leaderX = ego.X + 10^3;
% For non lane changing vehicles, the leader is whoever is longitudinally
% closer and with any part of the body in the same lane.
% 1.8m (half lane) + 0.9m (half veh width)
for n = 1:nv
    if allVehicles(n).X > ego.X
        if abs(allVehicles(n).Y - ego.Y) <= 2.7 ...
                && allVehicles(n).X < leaderX
            leaderIdx = n;
            leaderX = allVehicles(n).X;
        end
    end
end

== matlab function full_maneuver_platoon/Ld/CACC origin lane/Controller Real Leader/switch free flow/MATLAB Function ==
  data: h input; maxGap output; d0 input; vRef input; ev input; ehDot input; ea input; Kp parameter; Kd parameter; Ka parameter; Kdd parameter
function maxGap = followingGapThreshold(h, d0, vRef, ev, ehDot, ea, Kp, Kd, Ka, Kdd)

maxGap = h*vRef + d0 - 1/Kp*(Kd*ev + Kdd*ehDot + Ka*ea);

== stateflow chart full_maneuver_platoon/Fd/Lane Change Strategy/Strategy 1: synchronous/Chart ==
  state generatingGapForMergingVehicle
    entry:
    maneuverState = 1;
    hasVirtualLeader = true;
  state laneKeeping
    entry:
    maneuverState = 0;
    % canStartLaneChange = false;
  state gapClosing
    entry:
    maneuverState = 5;
    mustIncreaseGap = false;
  state generatingGap
    entry:
    maneuverState = 1;
    mustIncreaseGap = true;
    if positionInPlatoon == 1
    hasVirtualLeader = true;
    end
    if positionInPlatoon == length(platoonStates)
    hasVirtualFollower = true;
    end
  state waitingForGapClosing
    entry:
    maneuverState = 4;
    hasVirtualLeader = false;
  state laneChanging
    entry:
    maneuverState = 3;
    canStartLaneChange = true;
    hasVirtualFollower = false;
  state waitingForPlatoonSafeGap
    entry:
    maneuverState = 2;
  (default) -> laneKeeping
  laneKeeping -> generatingGapForMergingVehicle [order 1] : [gapRequest && platoonStates(end) <= 3]
  generatingGapForMergingVehicle -> laneKeeping : [platoonStates(end) > 3]
  gapClosing -> laneKeeping : [isGapClosed...
      | || (positionInPlatoon == 1 ...
      | && platoonStates(positionInPlatoon + 1) == 0)]
  waitingForGapClosing -> gapClosing : [positionInPlatoon == length(platoonStates) || ...
      | platoonStates(positionInPlatoon + 1) == 0]
  laneKeeping -> generatingGap [order 2] : [hasLaneChangeIntention && ~isLaneChangeDone ...
      |  && ((positionInPlatoon == 1) || (platoonStates(positionInPlatoon - 1)>1))]
  laneChanging -> waitingForGapClosing : [isLaneChangeDone]
  generatingGap -> waitingForPlatoonSafeGap : [isLaneChangeSafe]
  waitingForPlatoonSafeGap -> laneChanging : [platoonStates(end)>1]
  data: gapRequest input; hasLaneChangeIntention input; maneuverState output uint8 =uint8(0); mustIncreaseGap output =false; positionInPlatoon input; platoonStates input; isLaneChangeDone input; isLaneChangeSafe input; canStartLaneChange output =false; hasVirtualLeader output =false; hasVirtualFollower output =false; isGapClosed input

== matlab function full_maneuver_platoon/Fd/Lane Change Strategy/Strategy 1: synchronous/determine virtual leader idx/determineVirtualLeader ==
  data: nVehicles input; lcFlag input; virtualLeaderIdx output
function virtualLeaderIdx  = ...
    determineVirtualLeader(nVehicles, lcFlag)

% Strategy 'synchronous': all vehicles move together when gap fits the
% whole platoon
% Important assumption:
% The array of vehicles is ordered as [Ld, Fd, Lo, p1, ..., pN, Fo]

if ~lcFlag % gap generating vehicle
    virtualLeaderIdx = nVehicles-1; % last platoon vehicle
else % lane changing vehicle
    virtualLeaderIdx = 1;
end

end

== stateflow chart full_maneuver_platoon/Fd/Lane Change Strategy/Strategy 2: leader first/Chart ==
  state laneKeeping
    entry:
    maneuverState = 0;
    % canStartLaneChange = false;
  state generatingGapForMergingVehicle
    entry:
    maneuverState = 1;
    hasVirtualLeader = true;
  state gapClosing
    entry:
    maneuverState = 5;
    mustIncreaseGap = false;
  state waitingLeaderLaneChange
    entry:
    maneuverState = 1;
    hasVirtualLeader = true;
  state waitingForGapClosing
    entry:
    maneuverState = 4;
    hasVirtualLeader = false;
  state laneChanging
    entry:
    maneuverState = 3;
    canStartLaneChange = true;
    hasVirtualFollower = false;
  state generatingGap
    entry:
    maneuverState = 2;
    mustIncreaseGap = true;
    hasVirtualLeader = true;
    hasVirtualFollower = true;
  (default) -> laneKeeping
  laneKeeping -> generatingGapForMergingVehicle [order 2] : [gapRequest && platoonStates(end) <= 3]
  gapClosing -> laneKeeping : [isGapClosed...
      | || (positionInPlatoon == 1 ...
      | && sum(platoonStates(2:end)) == 0)]
  generatingGapForMergingVehicle -> laneKeeping : [platoonStates(end) > 3]
  laneKeeping -> waitingLeaderLaneChange [order 1] : [hasLaneChangeIntention && ~isLaneChangeDone ...
      |  && (positionInPlatoon == 1 || platoonStates(positionInPlatoon - 1) > 1)]
  waitingForGapClosing -> gapClosing : [true]
  waitingLeaderLaneChange -> generatingGap : [positionInPlatoon == 1 || platoonStates(positionInPlatoon - 1) > 4]
  laneChanging -> waitingForGapClosing : [isLaneChangeDone]
  generatingGap -> laneChanging : [isLaneChangeSafe]
  data: gapRequest input; hasLaneChangeIntention input; maneuverState output uint8 =uint8(0); mustIncreaseGap output =false; positionInPlatoon input; platoonStates input; isLaneChangeDone input; isLaneChangeSafe input; canStartLaneChange output =false; hasVirtualLeader output =false; hasVirtualFollower output =false; isGapClosed input
